simulink model "Bahnplanung_lauffaehig_auf_Robotino"  (R2015b)
settings: Solver=ode3  StartTime=0.0  StopTime=inf  FixedStep=0.005  RelTol=1e-3
undefined symbols (not defined in the file or in its folder): Com1, none
libraries: xpcobsoletelib x4, xpcrtudplib x3, simulink x2, xpcseriallib x1, slrtlib x1
(part 2 of 2)

== matlab function Bahnplanung_lauffaehig_auf_Robotino/Bahnplanung/Ausweichmanoever ==
  data: RobotinoPos input; StoerPos input; Vektor input; Ausweich output
function Ausweich  = fcn(RobotinoPos, StoerPos, Vektor)
Abstand=zeros([2 4]);
Ausweich=zeros([2 4]);%Zeile1 =Richtung(winkel in Rad) Zeile2=Intensität
for i=1:4
    Abstand(1,i)=RobotinoPos(1)-StoerPos(1+((i-1)*3));
    Abstand(2,i)=RobotinoPos(2)-StoerPos(2+((i-1)*3));
    Hyp=sqrt(Abstand(1,i)^2+Abstand(2,i)^2);
    if Hyp <=1000
        if Abstand(1,i) >= 0
             Ausweich(1,i)=+asin(Abstand(2,i)/Hyp)-pi/2;
        else
            Ausweich(1,i)=-asin(Abstand(2,i)/Hyp)+pi/2;
        end
        HypZiel=sqrt(Vektor(1)^2+Vektor(2)^2);
         if Vektor(1) >= 0
            Fahrwinkel=+asin(Vektor(2)/HypZiel);
        else
            Fahrwinkel=-asin(Vektor(2)/HypZiel+pi);
        end
        if (Fahrwinkel-(Ausweich(1,i)+pi/2) <= pi/2)&& (Fahrwinkel-(Ausweich(1,i)+pi/2)  >= -pi/2)
            Ausweich(2,i)=1;
        else
           Ausweich(2,i)=0; 
        end
       
%         if (Vektor(2)~=0) && (sin(Ausweich(1,i)+pi/2)~=0)
%             Ausweich(2,i)=Vektor(2)/sin(Ausweich(1,i)+pi/2);
%         elseif (Vektor(1)~=0)&&(cos(Ausweich(1,i)+pi/2)~=0)
%              Ausweich(2,i)=Vektor(1)/cos(Ausweich(1,i)+pi/2);
%         else
%              Ausweich(2,i)=0;
%         end
    else
        Ausweich(1,i)=0;
        Ausweich(2,i)=0;
    end
end

== matlab function Bahnplanung_lauffaehig_auf_Robotino/Bahnplanung/IR_Daten_Erfassen ==
  data: RobotinoDaten input; IRWerte output; RobPos input
function IRWerte = fcn(RobotinoDaten,RobPos)
IRWerte=zeros([2 9]);
IRDaten=zeros([1 9]);
IRDaten=RobotinoDaten(6:14);

for x=1:9
    if  (isnan(IRDaten(x))==0) && (IRDaten(x) <= 300)
    IRWerte(1,x)=cos(((x-1)*40*pi/180)+RobPos(3))*(IRDaten(x)+200)+RobPos(1);
    IRWerte(2,x)=sin(((x-1)*40*pi/180)+RobPos(3))*(IRDaten(x)+200)+RobPos(2);
    else
    IRWerte(1,x)=NaN;
    IRWerte(2,x)=NaN;
    end
end

== stateflow chart Bahnplanung_lauffaehig_auf_Robotino/Bahnplanung/Fifo ==
  settings: updateMethod=DISCRETE  sampleTime=0.005
  state FIFOStationen
    state Auftrag_Roboter_1
    state Zielbereich_untersuchen
      entry:
      ersterFifo=floor(Zielstation/2)*3+2*mod(Zielstation,2)+1;
    state Fifo_einfachbesetzt1
      entry:
      zweiterFifo=floor(Zielstation/2)*3+1+1;
      Fifo=2;
    state Fifo_frei
      entry:
      Fifo=1;
    state Fifo_doppelt_besetzt
      entry:
      dritterFifo=floor(Zielstation/2)*3+2-2*mod(Zielstation,2)+1;
      Fifo=3;
    state Fifo_voll
      entry:
      Fifo=4;
    state Uebergabepunkt_gleich_Zielpunkt
      entry:
      Fifo=0;
    (default) -> Auftrag_Roboter_1
    Auftrag_Roboter_1 -> Zielbereich_untersuchen : [Zielposition>-1]
    Zielbereich_untersuchen -> Fifo_einfachbesetzt1 [order 1] : [(FifoArray(ersterFifo)~=0)| (FifoArray(ersterFifo)==0 & StationArray(Zielstation+1)~=0) ]
    Uebergabepunkt_gleich_Zielpunkt -> Zielbereich_untersuchen
    Zielbereich_untersuchen -> Uebergabepunkt_gleich_Zielpunkt [order 2]
    Fifo_einfachbesetzt1 -> Fifo_frei [order 2] : [FifoArray(ersterFifo)==0]
    Fifo_einfachbesetzt1 -> Fifo_doppelt_besetzt [order 1] : [(FifoArray(zweiterFifo)~=0)]
    Fifo_doppelt_besetzt -> Fifo_voll [order 2] : [(FifoArray(dritterFifo)~=0)]
    Fifo_frei -> Uebergabepunkt_gleich_Zielpunkt : [ StationArray(Zielstation+1)==0]
    Fifo_doppelt_besetzt -> Fifo_einfachbesetzt1 [order 1] : [FifoArray(zweiterFifo)==0]
    Fifo_voll -> Fifo_doppelt_besetzt : [FifoArray(dritterFifo)==0]
  state Wartebereich
    entry: Fifo=4;
  state Ladestation
    entry: Fifo=0;
  (default) -> Wartebereich
  Wartebereich -> FIFOStationen [order 1] : [Zielstation<8]
  FIFOStationen -> Wartebereich [order 1] : [Zielstation==10]
  Ladestation -> Wartebereich [order 1] : [Zielstation==10]
  Wartebereich -> Ladestation [order 2] : [Zielstation>=8 & Zielstation<10]
  Ladestation -> FIFOStationen [order 2] : [Zielstation<8]
  FIFOStationen -> Ladestation [order 2] : [Zielstation>=8 & Zielstation<10]
  data: FifoArray input; Zielposition input; Zielstation input; Fifo output; StationArray input; dritterFifo local; zweiterFifo local; ersterFifo local

== stateflow chart Bahnplanung_lauffaehig_auf_Robotino/Bahnplanung/Kommunikation_mit_GW1_3 ==
  state KommunikationGW3
    state Fertigungsbereich
      entry:Transportbereich=0,
      Fertigungsbereich=1;
      state RFID_einchecken
        entry:Zielposition=Ziel-mod(Ziel,10)+3,
        Aktion_an_Position=Aktion_Warten,
        Status=2;
      state Startpunkt
        entry: Zielposition=Ziel-mod(Ziel,10);
        Aktion_an_Position=Aktion_Warten,
        Status=1;
      state Warten
        entry: BereichVerlassen=1,
        if  Werkstueck==0
        Status=0;
        end
      state Position_anfahren
        entry:Zielposition=Ziel,
        Status=1,
        if Werkstueck==0
        Aktion_an_Position=Aktion_Aufnehmen;
        else
        Aktion_an_Position=Aktion_Ablegen;
        end
      state Bereich_verlassen
        entry:Zielposition=Ziel-mod(Ziel,10)+4,
        Aktion_an_Position=Aktion_Warten,
        Status=1;
      state RFID_auschecken
        entry:Zielposition=Ziel-mod(Ziel,10)+3,
        Aktion_an_Position=Aktion_Warten,
        Status=3;
      Startpunkt -> RFID_einchecken [order 1] : [Ziel_anfordern & Werkstueck==1]
      (default) -> Startpunkt
      RFID_einchecken -> Position_anfahren : [RFID_Anmeldung==1]
      Startpunkt -> Position_anfahren [order 2] : [Ziel_anfordern & Werkstueck==0]
      Bereich_verlassen -> Warten : Ziel_anfordern
      Position_anfahren -> Bereich_verlassen [order 2] : [Ziel_anfordern & (Aktion_an_Position==Aktion_Ablegen)]
      Position_anfahren -> RFID_auschecken [order 1] : [Ziel_anfordern & (Aktion_an_Position==Aktion_Aufnehmen)]
      RFID_auschecken -> Bereich_verlassen : [RFID_Abmeldung==1]
    state Transportbereich
      entry:Transportbereich=1,
      Fertigungsbereich=0,
      BereichVerlassen=0;
    state Init
      entry: Transportbereich=1,
      Fertigungsbereich=0,
      Status=0;
    (default) -> Init
    Transportbereich -> Fertigungsbereich : ZielStation_Erreicht
    Init -> Transportbereich
    Fertigungsbereich -> Transportbereich : [BereichVerlassen==1]
  data: Transportbereich output; Fertigungsbereich output; Ziel input; Zielposition output; Aktion_an_Position output; Aktion_Warten local double =2; Aktion_Aufnehmen local double =1; Aktion_Ablegen local double =0; Werkstueck input double; Wartezeit local double =5; RFID_Anmeldung input; RFID_Abmeldung input; BereichVerlassen local; Status output
  events: Ziel_anfordern input RISING_EDGE_EVENT; ZielStation_Erreicht input RISING_EDGE_EVENT

== matlab function Bahnplanung_lauffaehig_auf_Robotino/Bahnplanung/Globale Markierung ==
  data: Robbi input; FifoArray input; FifoArray1 output; StationArray1 output; LadeArray input; LadeArray1 output
function [FifoArray1,StationArray1,LadeArray1]= fcn(Robbi,FifoArray,LadeArray)
X=zeros([1 4]);
Y=zeros([1 4]);
X=[Robbi(1) Robbi(4) Robbi(7) Robbi(10)];
Y=[Robbi(2) Robbi(5) Robbi(8) Robbi(11)];
FifoArray1=zeros([1 12]);
FifoArray1=FifoArray(1:12);
StationArray1=zeros([1 8]);
LadeArray1=zeros([1 2]);
LadeArray1=LadeArray(1:2);
N=zeros([1 4]);
S=zeros([1 4]);
L=zeros([1 4]);
for n= 1 : 1 : 4
    L(n)=round((Y(n)-2592)/500)+1;
    N(n)=round((X(n)-703)/400)+1;   % Berechnung in welchem Fifo der Roboter sich befindet
    S(n)=round((X(n)-900)/560)+1;   %Berechnung in welcher Station der Roboter sich befindet
     if (X(n)<=6000 || X(n)>6500)
        for i=1:2
            if LadeArray1(i)==n
                LadeArray1(i)=0;
            end
        end
     end
    if (X(n)>6000 && X(n)<=6500 && Y(n)>2300 &&Y(n)<=3300)
        LadeArray1(L(n))=n;
    end  
   
    for i=1:8
          if StationArray1(i)==n
                StationArray1(i)=0;
            end
    end
    if (Y(n)>2100 && X(n)<5100) && S(n)<=8
         for i=1:12
            if FifoArray1(i)==n
                FifoArray1(i)=0;
            end
         end
       
        StationArray1(S(n))=n;
        
    else if (Y(n)<450 && (X(n)>100 && X(n)<5250))
        for i=1:12
            if FifoArray1(i)==n
                FifoArray1(i)=0;
            end
        end
            FifoArray1(N(n))=n;
        end
    end
end

== matlab function Bahnplanung_lauffaehig_auf_Robotino/Bahnplanung/MATLAB Function ==
  data: Vektor_In input; Vektor output; Transportbereich_aktiv input
function Vektor = fcn(Vektor_In,Transportbereich_aktiv)
Vektor=zeros([1 2]);
if Transportbereich_aktiv==1
    Vektor=Vektor_In;
end

== matlab function Bahnplanung_lauffaehig_auf_Robotino/Bahnplanung/Positionen_Robotinos_Filtern ==
  data: UDPDaten input; RobPos output; RobotinoID input; StoerPos output
function [RobPos,StoerPos]      = fcn(UDPDaten , RobotinoID)
StoerPos=zeros([1 15]);
RobPos=zeros([1 3]);
%     case 5
%         RobPos(1:3) = UDPDaten(13:15);
%         StoerPos(1:12)=UDPDaten(1:12);
 if RobotinoID == 4
        RobPos(1:3) = UDPDaten(10:12);
        StoerPos(1:9)=UDPDaten(1:9);
        %  StoerPos(10:12)=UDPDaten(13:15);
    elseif RobotinoID == 3
        RobPos(1:3) = UDPDaten(7:9);
        StoerPos(1:6)=UDPDaten(1:6);
        StoerPos(7:9)=UDPDaten(10:12);%      StoerPos(7:12)=UDPDaten(10:15);
    elseif RobotinoID == 2
        RobPos(1:3) = UDPDaten(4:6);
        StoerPos(1:3)=UDPDaten(1:3);
        StoerPos(4:9)=UDPDaten(7:12);%     StoerPos(4:12)=UDPDaten(7:15);
        elseif RobotinoID == 1
        RobPos(1:3) = UDPDaten(1:3);
        StoerPos(1:9)=UDPDaten(4:12);%     StoerPos(1:12)=UDPDaten(4:15);
end

== matlab function Bahnplanung_lauffaehig_auf_Robotino/Bahnplanung/Positionszuweisung ==
  data: Fifo input; Zielstation input; Endposition output; RoboterID input
function Endposition = fcn(Fifo,Zielstation,RoboterID)
Endposition=zeros([1 2]);

WartepositionX= 6311;
WartepositionY=[550 950 1350 1750 2150];

StationvorneX=[853 1361 2058 2559 3256 3762 4448 4953 6311 6311];
StationvorneY=[2300 2300 2300 2300 2300 2300 2300 2300 2592 3080];
%Stationhinten=[856 1364 2059 2560 3259 3763 4451 4958];

ersterFifo=floor(Zielstation/2)*3+2*mod(Zielstation,2);
zweiterFifo=floor(Zielstation/2)*3+1;
dritterFifo=floor(Zielstation/2)*3+2-2*mod(Zielstation,2);

if Fifo==0
    Endposition(1)=StationvorneX(Zielstation+1);
    Endposition(2)=StationvorneY(Zielstation+1);
    else if Fifo==1
        Endposition(1)= ersterFifo*400+703;
        Endposition(2)= 250;
       
    else if Fifo==2
            Endposition(1)= zweiterFifo*400+703;
            Endposition(2)= 250;
        
    else if Fifo==3
            Endposition(1)= dritterFifo*400+703;
            Endposition(2)= 250;
            else
            Endposition(2)= WartepositionY(RoboterID);
            Endposition(1)= WartepositionX;
        end
        end
        end
end
end

== matlab function Bahnplanung_lauffaehig_auf_Robotino/Bahnplanung/Vektorberechnung ==
  data: ZielPos input; Vektor output; RobotinoPos input; StoerPos input; IRWerte input; Zone output
function [Vektor,Zone] = fcn(ZielPos, RobotinoPos, StoerPos, IRWerte)
Stationen=[1103,2308,3507,4694,6300,6300;
            2832,2832,2832,2832,2608,3085;];
Vektor=zeros([1 2]);
%Stationen Einflussvektor
K=400;
sigma=187;
SVX=zeros([1 6]);
SVY=zeros([1 6]);
for x=1:6
SVX(x)= -K*exp(-((RobotinoPos(1)-Stationen(1,x))^2+(RobotinoPos(2)-Stationen(2,x))^2)/(2*(sigma^2)))*((RobotinoPos(1)-Stationen(1,x))/(sigma^2));
SVY(x)= -K*exp(-((RobotinoPos(1)-Stationen(1,x))^2+(RobotinoPos(2)-Stationen(2,x))^2)/(2*(sigma^2)))*((RobotinoPos(2)-Stationen(2,x))/(sigma^2));
end
%Zielvektor
K=0.3;%=0.3;

ZVX = K*(RobotinoPos(1)-ZielPos(1))/sqrt((RobotinoPos(1)-ZielPos(1))^2 +(RobotinoPos(2)-ZielPos(2))^2);
ZVY = K*(RobotinoPos(2)-ZielPos(2))/sqrt((RobotinoPos(1)-ZielPos(1))^2 +(RobotinoPos(2)-ZielPos(2))^2);

%Robtino Stoervektoren
%K=25 im Fifo
K=1000;%K=100;
sigma=224;
RVX=zeros([1 4]);
RVY=zeros([1 4]);
for x=1:4
RVX(x)=-K*exp(-((RobotinoPos(1)-StoerPos((x*3)-2))^2+(RobotinoPos(2)-StoerPos((x*3)-1))^2)/(2*(sigma^2)))*((RobotinoPos(1)-StoerPos((x*3)-2))/(sigma^2));
RVY(x)=-K*exp(-((RobotinoPos(1)-StoerPos((x*3)-2))^2+(RobotinoPos(2)-StoerPos((x*3)-1))^2)/(2*(sigma^2)))*((RobotinoPos(2)-StoerPos((x*3)-1))/(sigma^2));
end

%Infrarot Einflussvektor
K=500;
sigma=250;
IRVX=zeros([1 9]);
IRVY=zeros([1 9]);
for x=1:9
    if(isnan(IRWerte(1,x))==0)||(isnan(IRWerte(2,x))==0)
    %IRVX(x)=-K*exp(-((RobotinoPos(1)-IRWerte(1,x))^2+(RobotinoPos(2)-IRWerte(2,x))^2)/(2*(sigma^2)))*((RobotinoPos(1)-IRWerte(1,x))/(sigma^2));
    %IRVY(x)=-K*exp(-((RobotinoPos(1)-IRWerte(1,x))^2+(RobotinoPos(2)-IRWerte(2,x))^2)/(2*(sigma^2)))*((RobotinoPos(2)-IRWerte(2,x))/(sigma^2));
    IRVX=0;
    IRVY=0;
    else
    IRVX(x)=0;
    IRVY(x)=0;
    end
end


 
K=0.1; %Steigung der schrägen
x=RobotinoPos(1);
y=RobotinoPos(2);
x_test=0;
y_test=0;
VektorX=0;
VektorY=0;
 if (x >601) && (x<=5501) && (y>2501) && (y<=3201)
    Zone=4;
elseif (x >2751) && (x<=5501) && (y>3201)
    Zone=1;
elseif (x > 601) && (x<=2751) && (y>3201)
    Zone=2;
 elseif (x<=601) && (y>2501)
     Zone=3;
 else
     Zone=0;
 end
KE=100;
sigma=30;
 if Zone == 0 % Fahrbereich
     if (x <= 5500) && (y <= 2500)
         x_test=(1/sigma)*KE*exp(-x/sigma);
         y_test=(-1/sigma)*KE*exp((y-2500)/sigma);
     elseif (x > 5500) && (y <= 2500)
         x_test=(1/sigma)*KE*exp((-(x-5500)+(y-2500))/sigma);
         y_test=(-1/sigma)*KE*exp((-(x-5500)+(y-2500))/sigma);
     elseif (x > 5500) && (y > 2500)
         x_test=(1/sigma)*KE*exp(-(x-5500)/sigma);
         y_test=(-1/sigma)*KE*exp((y-3600)/sigma);
     end
 MVX=x_test+(-1/sigma)*KE*exp((x-7000)/sigma);
 MVY=y_test+(1/sigma)*KE*exp(-y/sigma);
 
 VektorX=sum(SVX(5:6))+sum(RVX)+ZVX+sum(IRVX)-MVX;
 VektorY=sum(SVY(5:6))+sum(RVY)+ZVY+sum(IRVY)-MVY;
 elseif Zone == 1 %Rinne nach rechts weg
     MVX=K; %Konstante Steigung
     MVY=-2*(y-3500)/10000; % Parabel abgeleitet
 VektorX=sum(RVX)-MVX;
 VektorY=sum(RVY)-MVY;
 elseif Zone == 2 %Rinne nach links weg
     MVX=-K; %Konstante Steigung
     MVY=-2*(y-3500)/10000; % Parabel abgeleitet
      VektorX=sum(RVX)-MVX;
      VektorY=sum(RVY)-MVY;
 elseif Zone == 3 %Rinne nach unten weg
     MVX=-2*(x-300)/10000; %Konstante Steigung
     MVY=-K; % Parabel abgeleitet
     VektorX=sum(RVX)+sum(IRVX)-MVX;
     VektorY=sum(RVY)+sum(IRVY)-MVY;
 else 
     MVX=0;
     MVY=K;
      VektorX=sum(RVX)+sum(SVY(1:4))-MVX;
      VektorY=sum(RVY)+sum(SVY(1:4))-MVY;
 end  
      Vektor(1)=VektorX;
      Vektor(2)=VektorY;
 end

== matlab function Bahnplanung_lauffaehig_auf_Robotino/Bahnplanung/ZielPosSplitten ==
  data: AktuellesZiel input; ZielPos output; Zielstation output
function [ZielPos,Zielstation]= fcn(AktuellesZiel)
ZielPos=mod(AktuellesZiel,10);
Zielstation=round(AktuellesZiel/10);

== matlab function Bahnplanung_lauffaehig_auf_Robotino/Bahnplanung/ZielStation_Erreicht ==
  data: Zielstation input; Erreicht output; AktuellePos input
function Erreicht = fcn(Zielstation , AktuellePos)
X=AktuellePos(1);
Y=AktuellePos(2);
S=round((X-900)/560);
if Y >2200 && Y<2500&& X>600 && X < 5200 && S==Zielstation
    Erreicht=1;
else
    Erreicht=0;
end

== matlab function Bahnplanung_lauffaehig_auf_Robotino/Trafo ==
  data: Vektor input; V_RobX output; Winkel input; V_RobY output
function [V_RobX, V_RobY]= fcn(Vektor,Winkel)
V_RobX=cos(Winkel)*Vektor(1)+sin(Winkel)*Vektor(2);
V_RobY=cos(Winkel)*Vektor(2)-sin(Winkel)*Vektor(1);

== matlab function Bahnplanung_lauffaehig_auf_Robotino/Begrenzung ==
  data: win input; wout output
function wout = fnc(win)
wert= zeros(1);
K=200;
if win > K
    wert = K;
elseif win <-K
    wert=-K;
else
    wert = win;
end
wout = wert;

== matlab function Bahnplanung_lauffaehig_auf_Robotino/Begrenzung1 ==
  data: win input; wout output
function wout = fnc(win)
wert= zeros(1);
K=200;
if win > K
    wert = K;
elseif win <-K
    wert=-K;
else
    wert = win;
end
wout = wert;

== matlab function Bahnplanung_lauffaehig_auf_Robotino/Bahnplanung/AusweichVektorBerechnung ==
  data: Vektor_In input; Vektor output; Ausweichwert input; Zone input; RobotinoPos input; ZielPos input
function Vektor = fcn(Vektor_In,Ausweichwert,Zone,RobotinoPos,ZielPos)
Vektor=zeros([1 2]);
%Ausweichmanöver

K=0.3;
AVX=zeros([1 4]);
AVY=zeros([1 4]);
 for x=1:4
 AVX(x)=K*Ausweichwert(2,x)*cos(Ausweichwert(1,x));
 AVY(x)=K*Ausweichwert(2,x)*sin(Ausweichwert(1,x));
 end
if Zone==0
 VektorX=Vektor_In(1)+sum(AVX);
 VektorY=Vektor_In(2)+sum(AVY);
else
 VektorX=Vektor_In(1);
 VektorY=Vektor_In(2);
end

%Bremsen vor dem Ziel
Distanz=sqrt((RobotinoPos(1)-ZielPos(1))^2+(RobotinoPos(2)-ZielPos(2))^2);
MaxDis=300;
if Distanz > MaxDis
Vektor(1) = VektorX;
Vektor(2) = VektorY;
else
Vektor(1) = VektorX*Distanz/MaxDis;
Vektor(2) = VektorY*Distanz/MaxDis;  
end

end
